simulink model "BLDC_Controller1"  (R2021a)
settings: Solver=FixedStepDiscrete  StartTime=0.0  StopTime=10  FixedStep=1e-05  RelTol=1e-3
libraries: simulink x18
settings Model: Creator=Deepak  LastModifiedBy=Hossam
settings SolverCC: AlgebraicLoopSolver=TrustRegion
settings DataIOCC: SaveOutput=off  SaveTime=off
settings OptimizationCC: DefaultParameterBehavior=Inlined  UseDivisionForNetSlopeComputation=on  GainParamInheritBuiltInType=on  UseFloatMulNetSlope=on  InlineInvariantSignals=on  PassReuseOutputArgsAs=Individual arguments  ZeroExternalMemoryAtStartup=off  ZeroInternalMemoryAtStartup=off  NoFixptDivByZeroProtection=on  EfficientFloat2IntCast=on  LifeSpan=1  OptimizeBlockOrder=speed  DifferentSizesBufferReuse=on  EfficientTunableParamExpr=on
settings DebuggingCC: SignalInfNanChecking=error  SignalRangeChecking=error  ReadBeforeWriteMsg=EnableAllAsError  WriteAfterWriteMsg=EnableAllAsError  WriteAfterReadMsg=EnableAllAsError  AlgebraicLoopMsg=error  ArtificialAlgebraicLoopMsg=error  SaveWithDisabledLinksMsg=error  SaveWithParameterizedLinksMsg=error  BlockPriorityViolationMsg=error  SolverPrmCheckMsg=error  InheritedTsInSrcMsg=error  SingleTaskRateTransMsg=error  TasksWithSamePriorityMsg=error  SigSpecEnsureSampleTimeMsg=error  CheckMatrixSingularityMsg=error  IntegerOverflowMsg=error  ParameterUnderflowMsg=error  ParameterPrecisionLossMsg=error  ParameterTunabilityLossMsg=error  UnderSpecifiedDataTypeMsg=error  UnnecessaryDatatypeConvMsg=warning  VectorMatrixConversionMsg=error  SignalLabelMismatchMsg=error  UnconnectedInputMsg=error  UnconnectedOutputMsg=error  UnconnectedLineMsg=error  SFcnCompatibilityMsg=error  UniqueDataStoreMsg=error  BusObjectLabelMismatch=error  RootOutportRequireBusObject=error  AssertControl=DisableAll  ModelReferenceIOMsg=error  ModelReferenceIOMismatchMessage=error  UnknownTsInhSupMsg=error  ModelReferenceDataLoggingMessage=error  StateNameClashWarn=warning  StrictBusMsg=ErrorOnBusTreatedAsVector  NonBusSignalsTreatedAsBus=error  SFInvalidInputDataAccessInChartInitDiag=error  SFTransitionOutsideNaturalParentDiag=error  SFUnreachableExecutionPathDiag=error  SFUndirectedBroadcastEventsDiag=error  SFTransitionActionBeforeConditionDiag=error  SFTemporalDelaySmallerThanSampleTimeDiag=error  SFSelfTransitionDiag=error  SFExecutionAtInitializationDiag=error  IntegerSaturationMsg=error
settings HardwareCC: ProdBitPerPointer=32  ProdBitPerSizeT=32  ProdBitPerPtrDiffT=32  ProdLargestAtomicInteger=Long  ProdLargestAtomicFloat=Double  ProdWordSize=32  ProdLongLongMode=on  ProdHWDeviceType=ARM Compatible->ARM Cortex-M
settings SFSimCC: CompileTimeRecursionLimit=0  EnableRuntimeRecursion=off  MATLABDynamicMemAlloc=off  CustomCodeUndefinedFunction=UseInterfaceOnly
settings RTWCC: SystemTargetFile=ert.tlc  TemplateMakefile=ert_default_tmf  SILDebugging=on
settings CodeAppCC: ForceParamTrailComments=on  IgnoreCustomStorageClasses=off  OperatorAnnotations=on  SimulinkDataObjDesc=on  SFDataObjDesc=on  CustomSymbolStrGlobalVar=rt$N$M  CustomSymbolStrType=$N$M  CustomSymbolStrFcn=$N$M$F  CustomSymbolStrMacro=$N$M  InsertBlockDesc=on  ReqsInCode=on
settings ERTTargetCC: TargetLangStandard=C99 (ISO)  UtilityFuncGeneration=Shared location  GenerateSampleERTMain=on  IncludeMdlTerminateFcn=off  CombineSignalStateStructs=on  SuppressErrorStatus=on  SupportAbsoluteTime=off  CodeInterfacePackaging=Reusable function  SupportNonFinite=off  SupportComplex=off  ParenthesesLevel=Maximum  CastingMode=Standards  GenerateSharedConstants=off  InlinedParameterPlacement=NonHierarchical  ERTCustomFileTemplate=example_file_process.tlc  ERTFilePackagingFormat=CompactWithDataFile  EnableSignedLeftShifts=off  EnableSignedRightShifts=off

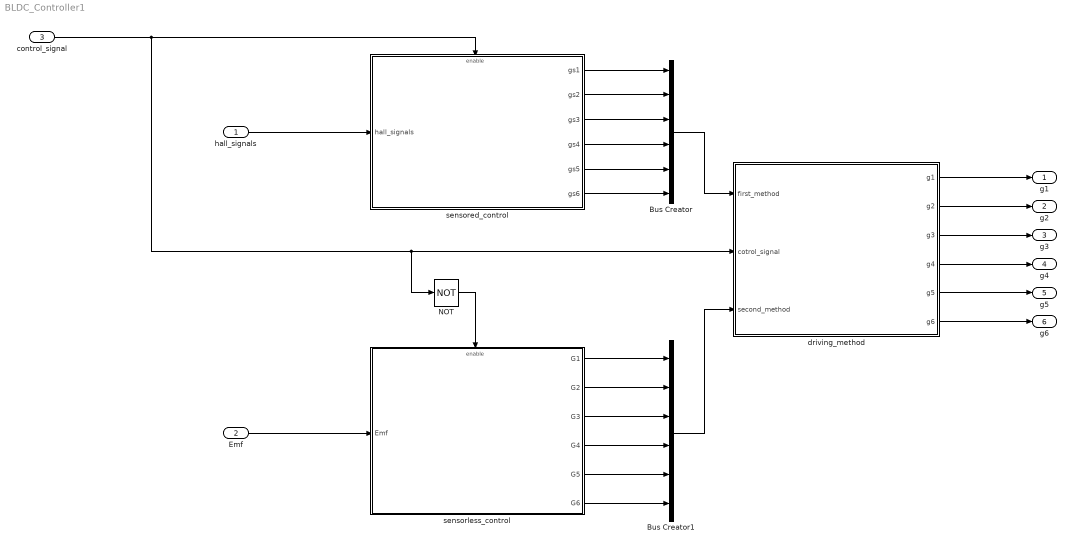
== system BLDC_Controller1 ==
  "hall_signals " : Inport  OutDataTypeStr=boolean  PortDimensions=3  SampleTime=[1.0000000000000001e-05,0]
  Emf : Inport  Port=2  OutDataTypeStr=double  PortDimensions=3  SampleTime=[1.0000000000000001e-05,0]
  control_signal : Inport  Port=3  OutDataTypeStr=boolean  PortDimensions=1  SampleTime=1e-5
  Bus Creator : BusCreator  Inputs=6
  Bus Creator1 : BusCreator  Inputs=6
  NOT : Logic  Operator=NOT  AllPortsSameDT=off  OutDataTypeStr=boolean
  driving_method : Subsystem
  sensored_control : Subsystem
  sensorless_control : Subsystem
  g1 : Outport  OutDataTypeStr=boolean  PortDimensions=1  SampleTime=[1.0000000000000001e-05,0]
  g2 : Outport  Port=2  OutDataTypeStr=boolean  PortDimensions=1  SampleTime=[1.0000000000000001e-05,0]
  g3 : Outport  Port=3  OutDataTypeStr=boolean  PortDimensions=1  SampleTime=[1.0000000000000001e-05,0]
  g4 : Outport  Port=4  OutDataTypeStr=boolean  PortDimensions=1  SampleTime=[1.0000000000000001e-05,0]
  g5 : Outport  Port=5  OutDataTypeStr=boolean  PortDimensions=1  SampleTime=[1.0000000000000001e-05,0]
  g6 : Outport  Port=6  OutDataTypeStr=boolean  PortDimensions=1  SampleTime=[1.0000000000000001e-05,0]
  wires:
  "hall_signals "/1 -> sensored_control/1("hall_signals ")
  Emf/1 -> sensorless_control/1(Emf)
  control_signal/1 -> driving_method/2(cotrol_signal), NOT/1, sensored_control/Enable
  sensored_control/1(gs1) -> Bus Creator/1
  sensored_control/2(gs2) -> Bus Creator/2
  sensored_control/3(gs3) -> Bus Creator/3
  sensored_control/4(gs4) -> Bus Creator/4
  sensored_control/5(gs5) -> Bus Creator/5
  sensored_control/6(gs6) -> Bus Creator/6
  sensorless_control/1(G1) -> Bus Creator1/1
  sensorless_control/2(G2) -> Bus Creator1/2
  sensorless_control/3(G3) -> Bus Creator1/3
  sensorless_control/4(G4) -> Bus Creator1/4
  sensorless_control/5(G5) -> Bus Creator1/5
  sensorless_control/6(G6) -> Bus Creator1/6
  driving_method/1(g1) -> g1/1
  driving_method/2(g2) -> g2/1
  driving_method/3(g3) -> g3/1
  driving_method/4(g4) -> g4/1
  driving_method/5(g5) -> g5/1
  driving_method/6(g6) -> g6/1
  Bus Creator/1 -> driving_method/1(first_method)
  Bus Creator1/1 -> driving_method/3(second_method)
  NOT/1 -> sensorless_control/Enable

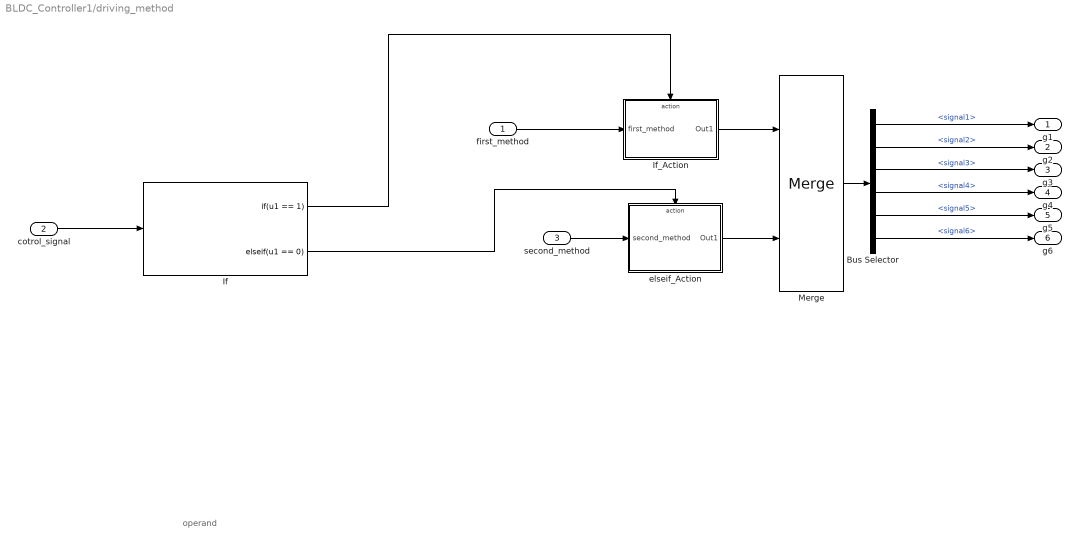
== system BLDC_Controller1/driving_method ==
  note: operand
  first_method : Inport
  cotrol_signal : Inport  Port=2
  second_method : Inport  Port=3
  Bus Selector : BusSelector  OutputSignals=signal1,signal2,signal3,signal4,signal5,signal6
  If : If  IfExpression=u1 == 1  ElseIfExpressions=u1 == 0  ShowElse=off
  If_Action : Subsystem  TreatAsAtomicUnit=on
  Merge : Merge
  elseif_Action : Subsystem  TreatAsAtomicUnit=on
  g1 : Outport
  g2 : Outport  Port=2
  g3 : Outport  Port=3
  g4 : Outport  Port=4
  g5 : Outport  Port=5
  g6 : Outport  Port=6
  wires:
  first_method/1 -> If_Action/1(first_method)
  If/1 -> If_Action/Action
  If/2 -> elseif_Action/Action
  second_method/1 -> elseif_Action/1(second_method)
  cotrol_signal/1 -> If/1
  elseif_Action/1(Out1) -> Merge/2
  If_Action/1(Out1) -> Merge/1
  Merge/1 -> Bus Selector/1
  Bus Selector/1 -> g1/1  "<signal1>"
  Bus Selector/2 -> g2/1  "<signal2>"
  Bus Selector/3 -> g3/1  "<signal3>"
  Bus Selector/4 -> g4/1  "<signal4>"
  Bus Selector/5 -> g5/1  "<signal5>"
  Bus Selector/6 -> g6/1  "<signal6>"

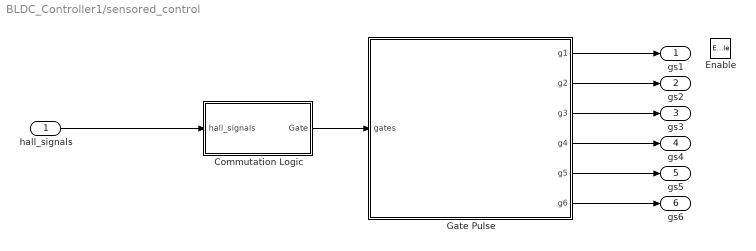
== system BLDC_Controller1/sensored_control ==
  "hall_signals " : Inport
  Enable : EnablePort
  Commutation Logic : Subsystem
  Gate Pulse : Subsystem
  gs1 : Outport
  gs2 : Outport  Port=2
  gs3 : Outport  Port=3
  gs4 : Outport  Port=4
  gs5 : Outport  Port=5
  gs6 : Outport  Port=6
  wires:
  Gate Pulse/5(g5) -> gs5/1
  Gate Pulse/3(g3) -> gs3/1
  Commutation Logic/1(Gate) -> Gate Pulse/1(gates)
  Gate Pulse/2(g2) -> gs2/1
  Gate Pulse/4(g4) -> gs4/1
  "hall_signals "/1 -> Commutation Logic/1("hall_signals ")
  Gate Pulse/1(g1) -> gs1/1
  Gate Pulse/6(g6) -> gs6/1

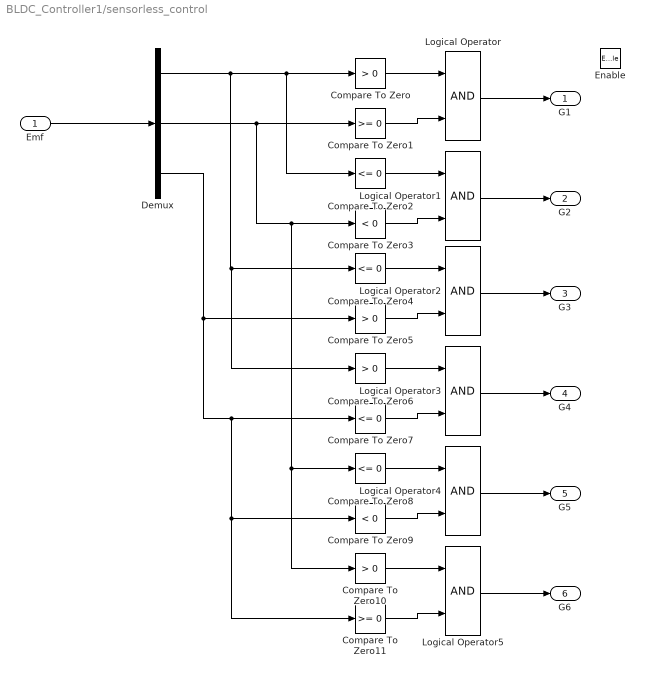
== system BLDC_Controller1/sensorless_control ==
  Emf : Inport
  Enable : EnablePort
  Compare To Zero{,5..6,10} (4 alike) : simulink/Logic and Bit Operations/Compare To Zero  relop=>  OutDataTypeStr=boolean
  Compare To Zero1 : simulink/Logic and Bit Operations/Compare To Zero  relop=>=  OutDataTypeStr=boolean
  Compare To Zero11 : simulink/Logic and Bit Operations/Compare To Zero  relop=>=  OutDataTypeStr=boolean
  Compare To Zero{2,4,7..8} (4 alike) : simulink/Logic and Bit Operations/Compare To Zero  relop=<=  OutDataTypeStr=boolean
  Compare To Zero3 : simulink/Logic and Bit Operations/Compare To Zero  relop=<  OutDataTypeStr=boolean
  Compare To Zero9 : simulink/Logic and Bit Operations/Compare To Zero  relop=<  OutDataTypeStr=boolean
  Demux : Demux  Outputs=3
  Logical Operator{,1..5} (6 alike) : Logic  AllPortsSameDT=off  OutDataTypeStr=boolean
  G1 : Outport
  G2 : Outport  Port=2
  G3 : Outport  Port=3
  G4 : Outport  Port=4
  G5 : Outport  Port=5
  G6 : Outport  Port=6
  wires:
  Compare To Zero10/1 -> Logical Operator5/1
  Compare To Zero3/1 -> Logical Operator1/2
  Demux/1 -> Compare To Zero6/1, Compare To Zero4/1, Compare To Zero2/1, Compare To Zero/1
  Compare To Zero9/1 -> Logical Operator4/2
  Demux/3 -> Compare To Zero9/1, Compare To Zero11/1, Compare To Zero7/1, Compare To Zero5/1
  Emf/1 -> Demux/1
  Demux/2 -> Compare To Zero1/1, Compare To Zero10/1, Compare To Zero8/1, Compare To Zero3/1
  Logical Operator/1 -> G1/1
  Compare To Zero11/1 -> Logical Operator5/2
  Logical Operator3/1 -> G4/1
  Logical Operator1/1 -> G2/1
  Compare To Zero8/1 -> Logical Operator4/1
  Compare To Zero1/1 -> Logical Operator/2
  Compare To Zero7/1 -> Logical Operator3/2
  Compare To Zero4/1 -> Logical Operator2/1
  Logical Operator2/1 -> G3/1
  Compare To Zero6/1 -> Logical Operator3/1
  Compare To Zero5/1 -> Logical Operator2/2
  Logical Operator4/1 -> G5/1
  Compare To Zero2/1 -> Logical Operator1/1
  Logical Operator5/1 -> G6/1
  Compare To Zero/1 -> Logical Operator/1

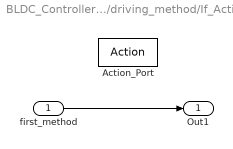
== system BLDC_Controller1/driving_method/If_Action ==
  first_method : Inport
  Action_Port : ActionPort  ActionPortLabel=if(u1 == 1)
  Out1 : Outport  VectorParamsAs1DForOutWhenUnconnected=off
  wires:
  first_method/1 -> Out1/1

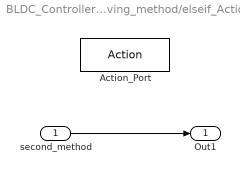
== system BLDC_Controller1/driving_method/elseif_Action ==
  second_method : Inport
  Action_Port : ActionPort  ActionPortLabel=elseif(u1 == 0)
  Out1 : Outport  VectorParamsAs1DForOutWhenUnconnected=off
  wires:
  second_method/1 -> Out1/1

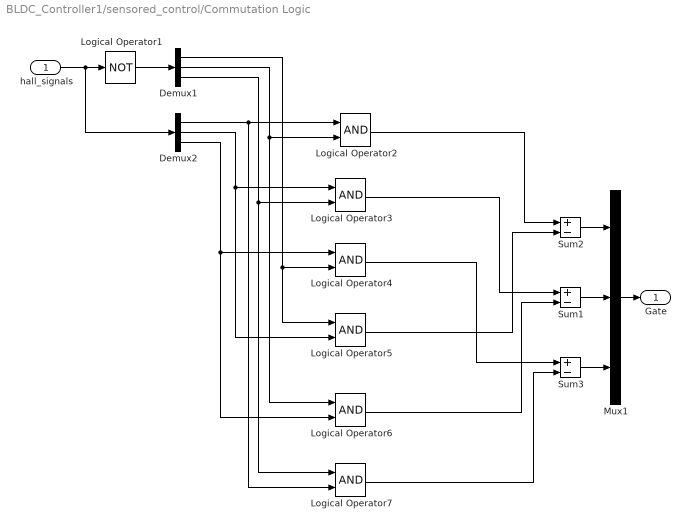
== system BLDC_Controller1/sensored_control/Commutation Logic ==
  "hall_signals " : Inport
  Demux1 : Demux  Outputs=3
  Demux2 : Demux  Outputs=3
  Logical Operator1 : Logic  Operator=NOT  AllPortsSameDT=off  OutDataTypeStr=boolean
  Logical Operator{2..7} (6 alike) : Logic  AllPortsSameDT=off  OutDataTypeStr=boolean
  Mux1 : Mux  Inputs=3
  Sum1 : Sum  Inputs=+-  OutDataTypeStr=double
  Sum2 : Sum  Inputs=+-  OutDataTypeStr=double
  Sum3 : Sum  Inputs=+-  OutDataTypeStr=double
  Gate : Outport  VectorParamsAs1DForOutWhenUnconnected=off
  wires:
  Demux2/1 -> Logical Operator7/2, Logical Operator2/1
  Demux1/3 -> Logical Operator7/1, Logical Operator3/2
  Demux2/2 -> Logical Operator3/1, Logical Operator5/2
  Sum1/1 -> Mux1/2
  Logical Operator3/1 -> Sum1/1
  "hall_signals "/1 -> Logical Operator1/1, Demux2/1
  Demux1/2 -> Logical Operator6/1, Logical Operator2/2
  Logical Operator2/1 -> Sum2/1
  Logical Operator7/1 -> Sum3/2
  Logical Operator4/1 -> Sum3/1
  Demux1/1 -> Logical Operator4/2, Logical Operator5/1
  Logical Operator6/1 -> Sum1/2
  Logical Operator5/1 -> Sum2/2
  Sum3/1 -> Mux1/3
  Logical Operator1/1 -> Demux1/1
  Mux1/1 -> Gate/1
  Sum2/1 -> Mux1/1
  Demux2/3 -> Logical Operator4/1, Logical Operator6/2

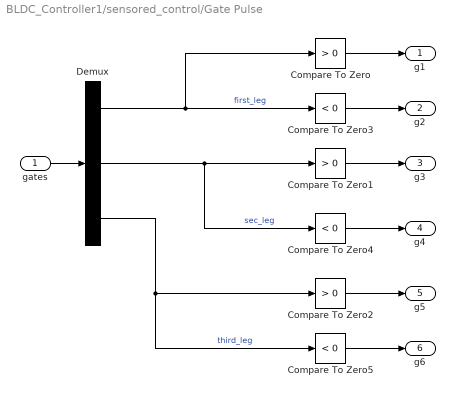
== system BLDC_Controller1/sensored_control/Gate Pulse ==
  gates : Inport
  Compare To Zero : simulink/Logic and Bit Operations/Compare To Zero  relop=>  OutDataTypeStr=boolean
  Compare To Zero1 : simulink/Logic and Bit Operations/Compare To Zero  relop=>  OutDataTypeStr=boolean
  Compare To Zero2 : simulink/Logic and Bit Operations/Compare To Zero  relop=>  OutDataTypeStr=boolean
  Compare To Zero3 : simulink/Logic and Bit Operations/Compare To Zero  relop=<  OutDataTypeStr=boolean
  Compare To Zero4 : simulink/Logic and Bit Operations/Compare To Zero  relop=<  OutDataTypeStr=boolean
  Compare To Zero5 : simulink/Logic and Bit Operations/Compare To Zero  relop=<  OutDataTypeStr=boolean
  Demux : Demux  Outputs=3
  g1 : Outport  VectorParamsAs1DForOutWhenUnconnected=off
  g2 : Outport  Port=2  VectorParamsAs1DForOutWhenUnconnected=off
  g3 : Outport  Port=3  VectorParamsAs1DForOutWhenUnconnected=off
  g4 : Outport  Port=4  VectorParamsAs1DForOutWhenUnconnected=off
  g5 : Outport  Port=5  VectorParamsAs1DForOutWhenUnconnected=off
  g6 : Outport  Port=6  VectorParamsAs1DForOutWhenUnconnected=off
  wires:
  Compare To Zero1/1 -> g3/1
  Demux/2 -> Compare To Zero4/1, Compare To Zero1/1  "sec_leg"
  Compare To Zero3/1 -> g2/1
  Demux/3 -> Compare To Zero5/1, Compare To Zero2/1  "third_leg"
  Compare To Zero2/1 -> g5/1
  Demux/1 -> Compare To Zero3/1, Compare To Zero/1  "first_leg"
  Compare To Zero4/1 -> g4/1
  Compare To Zero5/1 -> g6/1
  Compare To Zero/1 -> g1/1
  gates/1 -> Demux/1
